simulink model "SerialCom"  (R2020b)
settings: Solver=FixedStepDiscrete  StartTime=0.0  StopTime=inf  FixedStep=0.01  RelTol=1e-3
libraries: arduinolib x14, simulink x2, commutil2 x1, aerolibanimutils x1
settings Model: SimulationMode=external  ExtModeTrigDuration=2  Creator=Pablo  LastModifiedBy=Pablo
settings SolverCC: AutoInsertRateTranBlk=on
settings DataIOCC: ReturnWorkspaceOutputs=off
settings OptimizationCC: PassReuseOutputArgsAs=Individual arguments  MaxStackSize=64  EfficientTunableParamExpr=on
settings DebuggingCC: ParameterOverflowMsg=none  ParameterTunabilityLossMsg=error  ArithmeticOperatorsInVariantConditions=warning
settings HardwareCC: ProdBitPerInt=16  ProdBitPerPointer=16  ProdBitPerSizeT=16  ProdBitPerPtrDiffT=16  ProdLargestAtomicFloat=None  ProdWordSize=8  ProdHWDeviceType=Atmel->AVR  UseEmbeddedCoderFeatures=off  UseSimulinkCoderFeatures=off
settings SFSimCC: SimUseLocalCustomCode=off  MATLABDynamicMemAlloc=off  CustomCodeUndefinedFunction=UseInterfaceOnly
settings RTWCC: Description=Embedded Coder  SystemTargetFile=ert.tlc  HardwareBoard=Arduino Mega 2560  TemplateMakefile=ert_default_tmf  GenerateReport=on  RTWUseLocalCustomCode=off  Toolchain=Arduino AVR  BuildConfiguration=Faster Runs  IncludeHyperlinkInReport=on  LaunchReport=on  GenerateTraceInfo=on  GenerateTraceReport=on  GenerateTraceReportSl=on  GenerateTraceReportSf=on  GenerateTraceReportEml=on
settings CodeAppCC: ForceParamTrailComments=on  IgnoreCustomStorageClasses=off  OperatorAnnotations=on  SimulinkDataObjDesc=on  SFDataObjDesc=on  InsertBlockDesc=on
settings ERTTargetCC: SupportContinuousTime=on  SupportNonInlinedSFcns=on  SupportVariableSizeSignals=on

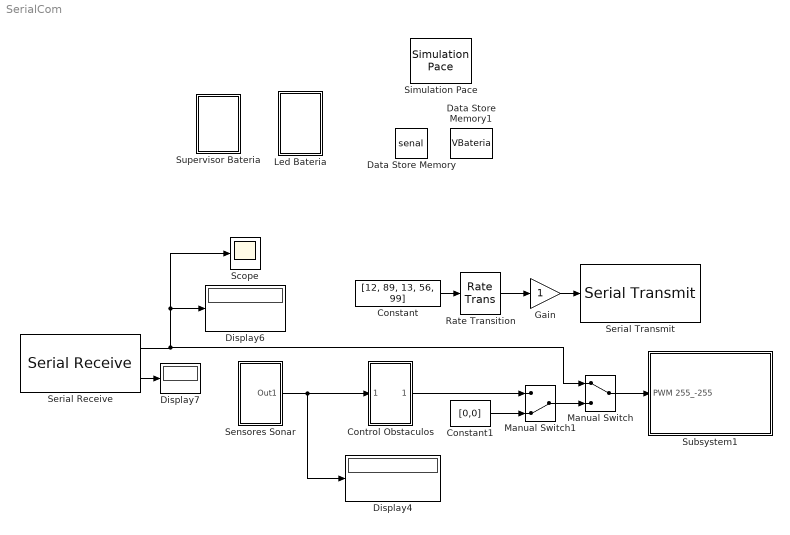
== system SerialCom ==
  Constant : Constant  Value=[12, 89, 13, 56, 99]
  Constant1 : Constant  Value=[0,0]
  Control Obstaculos : Subsystem
  Data Store Memory1 : DataStoreMemory  DataStoreName=VBateria  ReadBeforeWriteMsg=warning  WriteAfterWriteMsg=warning  WriteAfterReadMsg=warning  ShowAdditionalParam=off  OutDataTypeStr=double
  Data Store Memory : DataStoreMemory  DataStoreName=senal  ReadBeforeWriteMsg=warning  WriteAfterWriteMsg=warning  WriteAfterReadMsg=warning  ShowAdditionalParam=off
  Display4 : Display
  Display6 : Display
  Display7 : Display
  Gain : Gain  OutDataTypeStr=uint8
  Led Bateria : Subsystem
  Manual Switch : ManualSwitch
  Manual Switch1 : ManualSwitch  CurrentSetting=0
  Rate Transition : RateTransition  OutPortSampleTime=2
  Scope : Scope
  Sensores Sonar : Subsystem
  Serial Receive : arduinolib/Serial Receive  isARMArch=off  portNumber=3  DataType=uint8  Datalength=2  SampleTime=0.1  showOutStatus=on  blockPlatform=arduino
      settings: SourceProductBaseCode=ARDUINO
  Serial Transmit : arduinolib/Serial Transmit  portNumber=3  sendmode=write  sendformat=Decimal  floatprecision=2  blockPlatform=arduino
  Simulation Pace : aerolibanimutils/Simulation Pace  SimulationPace=1  SleepMode=MATLAB Thread  OutputPaceError=off  SampleTime=-1
  Subsystem1 : Subsystem
  Supervisor Bateria : Subsystem
  wires:
  Sensores Sonar/1(Out1) -> Control Obstaculos/1(In1), Display4/1
  Serial Receive/1 -> Scope/1, Display6/1, Manual Switch/1
  Serial Receive/2 -> Display7/1
  Manual Switch/1 -> Subsystem1/1(PWM 255_-255)
  Gain/1 -> Serial Transmit/1
  Rate Transition/1 -> Gain/1
  Constant/1 -> Rate Transition/1
  Manual Switch1/1 -> Manual Switch/2
  Control Obstaculos/1(PWM 255_-255) -> Manual Switch1/1
  Constant1/1 -> Manual Switch1/2

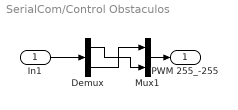
== system SerialCom/Control Obstaculos ==
  In1 : Inport
  Demux : Demux  Outputs=2
  Mux1 : Mux  Inputs=2
  PWM 255_-255 : Outport  VectorParamsAs1DForOutWhenUnconnected=off
  wires:
  Mux1/1 -> PWM 255_-255/1
  Demux/2 -> Mux1/1
  Demux/1 -> Mux1/2
  In1/1 -> Demux/1

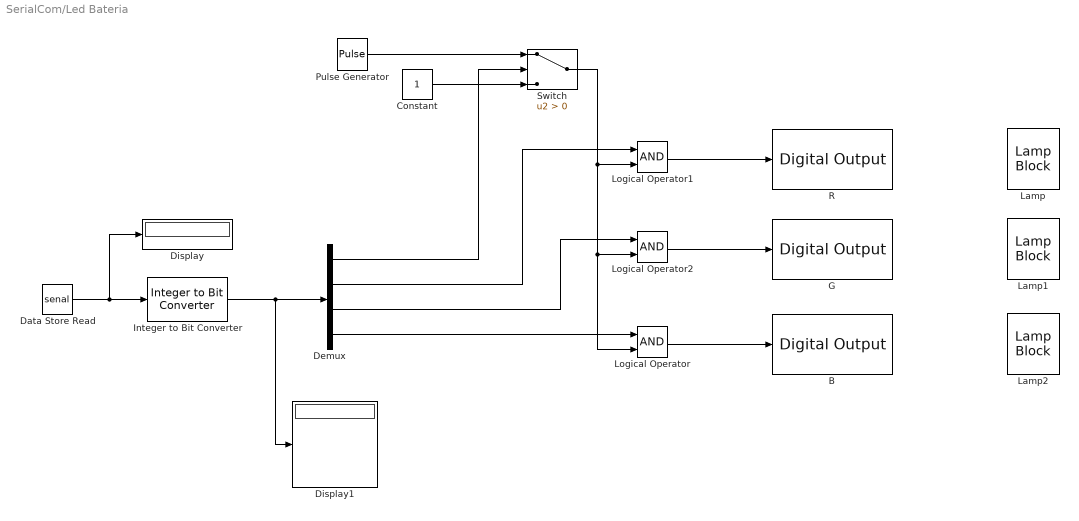
== system SerialCom/Led Bateria ==
  B : arduinolib/Digital Output  pinNumber=49  Direction=output  blockPlatform=arduino
  Constant : Constant
  Data Store Read : DataStoreRead  DataStoreName=senal
  Demux : Demux
  Display : Display
  Display1 : Display
  G : arduinolib/Digital Output  pinNumber=53  Direction=output  blockPlatform=arduino
  Integer to Bit Converter : commutil2/Integer to Bit Converter  nbits=4  signedInputValues=Unsigned  bitOrder=MSB first  outDtype=Inherit via internal rule
  Lamp : LampBlock
  Lamp1 : LampBlock
  Lamp2 : LampBlock
  Logical Operator : Logic  AllPortsSameDT=off  OutDataTypeStr=boolean
  Logical Operator1 : Logic  AllPortsSameDT=off  OutDataTypeStr=boolean
  Logical Operator2 : Logic  AllPortsSameDT=off  OutDataTypeStr=boolean
  Pulse Generator : DiscretePulseGenerator  PulseType=Time based  Period=1  PulseWidth=50
  R : arduinolib/Digital Output  pinNumber=51  Direction=output  blockPlatform=arduino
  Switch : Switch  Criteria=u2 > Threshold
  wires:
  Switch/1 -> Logical Operator/2, Logical Operator2/2, Logical Operator1/2
  Pulse Generator/1 -> Switch/1
  Demux/1 -> Switch/2
  Logical Operator/1 -> B/1
  Logical Operator1/1 -> R/1
  Logical Operator2/1 -> G/1
  Demux/4 -> Logical Operator/1
  Demux/3 -> Logical Operator2/1
  Demux/2 -> Logical Operator1/1
  Constant/1 -> Switch/3
  Integer to Bit Converter/1 -> Display1/1, Demux/1
  Data Store Read/1 -> Display/1, Integer to Bit Converter/1

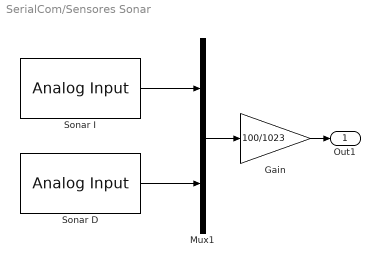
== system SerialCom/Sensores Sonar ==
  Gain : Gain  Gain=100/1023
  Mux1 : Mux  Inputs=2
  Sonar D : arduinolib/Analog Input  pinNumber=1  ReadResultsOnly=off  ConversionTriggerSource=Software  ExternalTriggerType=uint32( 0 )  OutputDataType=uint16  EnableConversionCompleteNotify=off  EnableOuputStatus=off  SampleTime=0.1  blockPlatform=arduino
  Sonar I : arduinolib/Analog Input  pinNumber=0  ReadResultsOnly=off  ConversionTriggerSource=Software  ExternalTriggerType=uint32( 0 )  OutputDataType=uint16  EnableConversionCompleteNotify=off  EnableOuputStatus=off  SampleTime=0.1  blockPlatform=arduino
  Out1 : Outport  VectorParamsAs1DForOutWhenUnconnected=off
  wires:
  Gain/1 -> Out1/1
  Mux1/1 -> Gain/1
  Sonar I/1 -> Mux1/1
  Sonar D/1 -> Mux1/2

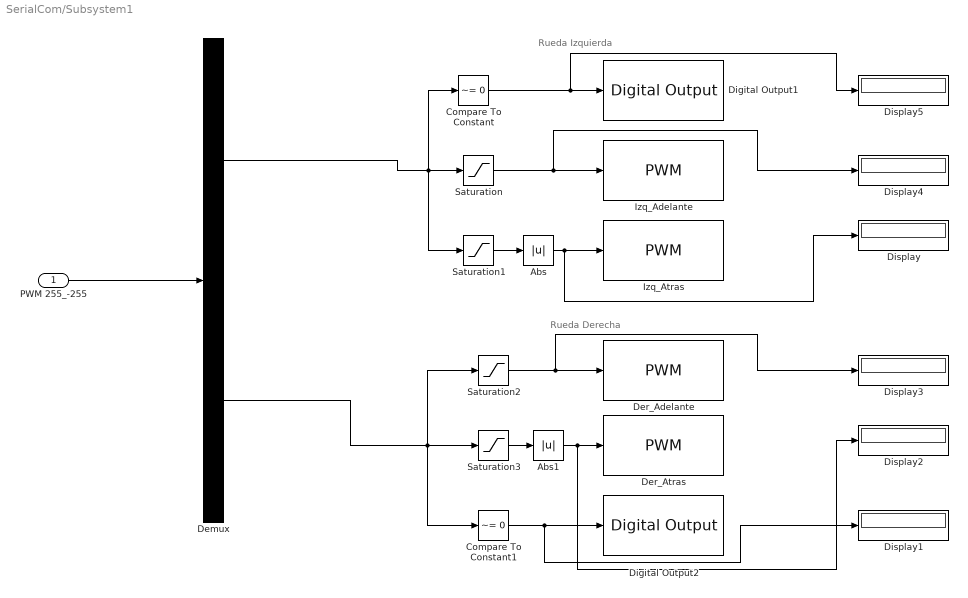
== system SerialCom/Subsystem1 ==
  note: Rueda Derecha
  note: Rueda Izquierda
  PWM 255_-255 : Inport
  Abs : Abs  OutDataTypeStr=uint8
  Abs1 : Abs  OutDataTypeStr=uint8
  Compare To Constant : simulink/Logic and Bit Operations/Compare To Constant  relop=~=  const=0  OutDataTypeStr=boolean
  Compare To Constant1 : simulink/Logic and Bit Operations/Compare To Constant  relop=~=  const=0  OutDataTypeStr=boolean
  Demux : Demux  Outputs=2
  Der_Adelante : arduinolib/PWM  pinNumber=8  frequencyType=Default  desiredFrequency=490.2  achievableFrequency=490.2
  Der_Atras : arduinolib/PWM  pinNumber=9  frequencyType=Default  desiredFrequency=490.2  achievableFrequency=490.2
  Digital Output1 : arduinolib/Digital Output  pinNumber=5  Direction=output  blockPlatform=arduino
  Digital Output2 : arduinolib/Digital Output  pinNumber=10  Direction=output  blockPlatform=arduino
  Display{,1..5} (6 alike) : Display
  Izq_Adelante : arduinolib/PWM  pinNumber=6  frequencyType=Default  desiredFrequency=490.2  achievableFrequency=490.2
  Izq_Atras : arduinolib/PWM  pinNumber=7  frequencyType=Default  desiredFrequency=490.2  achievableFrequency=490.2
  Saturation : Saturate  UpperLimit=255  LowerLimit=0
  Saturation1 : Saturate  UpperLimit=0  LowerLimit=-255  OutDataTypeStr=uint16
  Saturation2 : Saturate  UpperLimit=255  LowerLimit=0
  Saturation3 : Saturate  UpperLimit=0  LowerLimit=-255
  wires:
  Saturation/1 -> Display4/1, Izq_Adelante/1
  Compare To Constant/1 -> Display5/1, Digital Output1/1
  Saturation1/1 -> Abs/1
  PWM 255_-255/1 -> Demux/1
  Demux/1 -> Saturation1/1, Compare To Constant/1, Saturation/1
  Abs/1 -> Display/1, Izq_Atras/1
  Saturation3/1 -> Abs1/1
  Demux/2 -> Compare To Constant1/1, Saturation2/1, Saturation3/1
  Compare To Constant1/1 -> Display1/1, Digital Output2/1
  Abs1/1 -> Display2/1, Der_Atras/1
  Saturation2/1 -> Display3/1, Der_Adelante/1

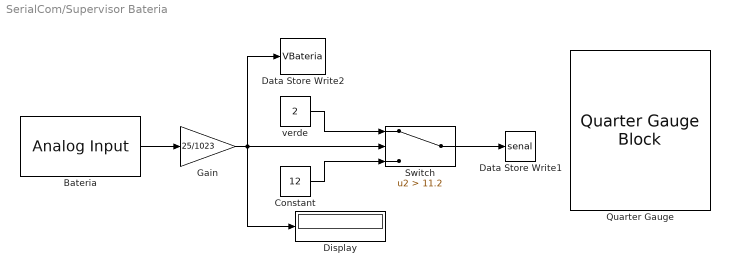
== system SerialCom/Supervisor Bateria ==
  "Bateria " : arduinolib/Analog Input  pinNumber=2  ReadResultsOnly=off  ConversionTriggerSource=Software  ExternalTriggerType=uint32( 0 )  OutputDataType=uint16  EnableConversionCompleteNotify=off  EnableOuputStatus=off  SampleTime=1  blockPlatform=arduino
  Constant : Constant  Value=12
  Data Store Write1 : DataStoreWrite  DataStoreName=senal
  Data Store Write2 : DataStoreWrite  DataStoreName=VBateria
  Display : Display
  Gain : Gain  Gain=25/1023  OutDataTypeStr=double
  Quarter Gauge : QuarterGaugeBlock  ScaleMin=10  ScaleMax=13
  Switch : Switch  Criteria=u2 > Threshold  Threshold=11.2  OutDataTypeStr=uint8
  verde : Constant  Value=2
  wires:
  "Bateria "/1 -> Gain/1
  Constant/1 -> Switch/3
  Gain/1 -> Switch/2, Display/1, Data Store Write2/1
  verde/1 -> Switch/1
  Switch/1 -> Data Store Write1/1
